simulink model "controller"  (R2019b)
settings: Solver=VariableStepAuto  StartTime=0.0  StopTime=10.0  RelTol=1e-3
settings Model: Creator=Avmash  LastModifiedBy=Avmash

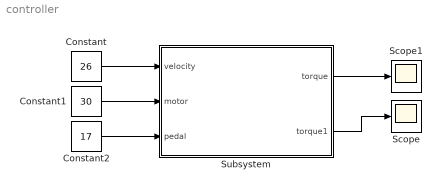
== system controller ==
  Constant : Constant  Value=26
  Constant1 : Constant  Value=30
  Constant2 : Constant  Value=17
  Scope : Scope
  Scope1 : Scope
  Subsystem : Subsystem
  wires:
  Constant/1 -> Subsystem/1(velocity)
  Constant1/1 -> Subsystem/2(motor)
  Subsystem/2(torque1) -> Scope/1
  Subsystem/1(torque) -> Scope1/1
  Constant2/1 -> Subsystem/3(pedal)

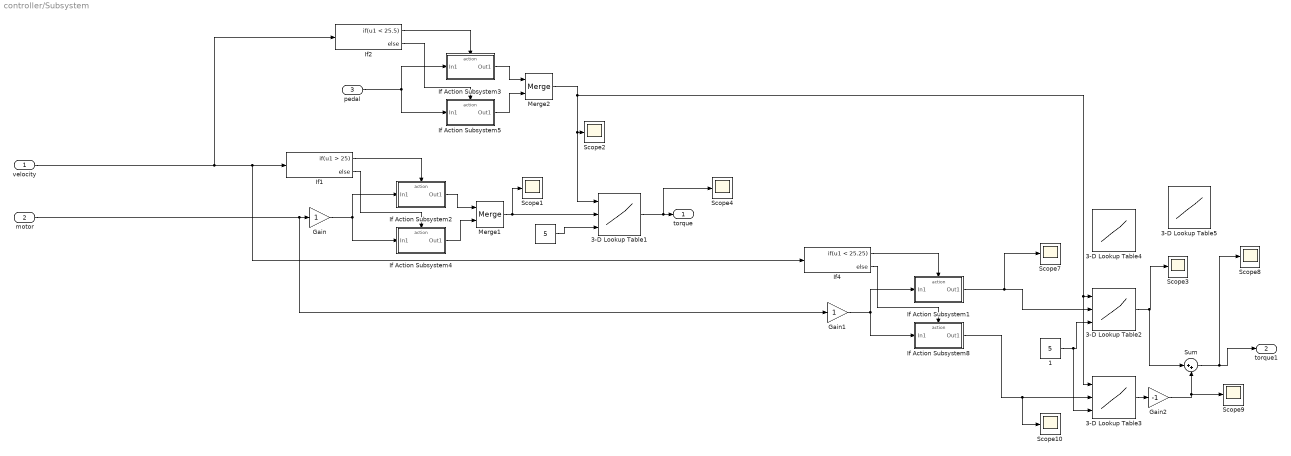
== system controller/Subsystem ==
  velocity : Inport
  motor : Inport  Port=2
  pedal : Inport  Port=3
  " " : Constant  Value=5
  " 1" : Constant  Value=5
  3-D Lookup Table1 : Lookup_n-D  NumberOfTableDimensions=3  BreakpointsForDimension1=[0,5,10,15,20]  BreakpointsForDimension2=[0,10,20,30,40]  BreakpointsForDimension3=[5, 7]  Table=reshape([0,5,10,15,20,0,10,15,20,25,0,10,20,25,30,0,10,20,30,35,0,10,20,30,40,0,5,10,15,20,0,10,15,20,25,0,10,20,25,30,0,10,20,30,35,0,10,20,30,40],5,5,2)  InternalRulePriority=Speed  RndMeth=Simplest  InputSameDT=on
  3-D Lookup Table2 : Lookup_n-D  NumberOfTableDimensions=3  BreakpointsForDimension1=[0,5,10,15,20]  BreakpointsForDimension2=[0,10,20,30,40]  BreakpointsForDimension3=[5, 7]  Table=reshape([0,5,10,15,20,0,10,15,20,25,0,10,20,25,30,0,10,20,30,35,0,10,20,30,40,0,5,10,15,20,0,10,15,20,25,0,10,20,25,30,0,10,20,30,35,0,10,20,30,40],5,5,2)  InternalRulePriority=Speed  RndMeth=Simplest  InputSameDT=on
  3-D Lookup Table3 : Lookup_n-D  NumberOfTableDimensions=3  BreakpointsForDimension1=[0,5,10,15,20]  BreakpointsForDimension2=[0,10,20,30,40]  BreakpointsForDimension3=[5, 7]  Table=reshape([0,0,0,0,0,0,10,15,20,25,0,10,20,25,30,0,10,20,30,35,0,10,20,30,40,0,5,10,15,20,0,10,15,20,25,0,10,20,25,30,0,10,20,30,35,0,10,20,30,40],5,5,2)  InternalRulePriority=Speed  RndMeth=Simplest  InputSameDT=on
  3-D Lookup Table4 : Lookup_n-D  NumberOfTableDimensions=3  BreakpointsForDimension1=[0,5,10,15,20]  BreakpointsForDimension2=[-40,-30,-20,-10,0,10,20,30,40]  BreakpointsForDimension3=[5, 7]  Table=reshape([0,-10,-20,-30,-40,0,-10,-20,-30,-35,0,-10,-20,-25,-30,0,-10,-15,-20,-25,0,5,10,15,20,0,10,15,20,25,0,10,20,25,30,0,10,20,30,35,0,10,20,30,40,0,-10,-20,-30,-40,0,-10,-20,-30,-35,0,-10,-20,-25,-30,0,-10,-15,-20,-25,0,5,10,15,20,0,10,15,20,25,0,10,20,25,30,0,10,20,30,35,0,10,20,30,40],5,9,2)  InternalRulePriority=Speed  RndMeth=Simplest  InputSameDT=on
  3-D Lookup Table5 : Lookup_n-D  NumberOfTableDimensions=3  BreakpointsForDimension1=[0,5,10,15,20]  BreakpointsForDimension2=[-40,-30,-20,-10,0]  BreakpointsForDimension3=[5, 7]  Table=|  InternalRulePriority=Speed  RndMeth=Simplest  InputSameDT=on
      | reshape([
      | 0,-10,-20,-30,-40,0,-10,-20,-30,-35,0,-10,-20,-25,-30,0,-10,-15,-20,-25,0,5,10,15,20,0,-10,-20,-30,-40,0,-10,-20,-30,-35,0,-10,-20,-25,-30,0,-10,-15,-20,-25,0,5,10,15,20],5,5,2)
  Gain : Gain
  Gain1 : Gain
  Gain2 : Gain  Gain=-1
  If Action Subsystem1 : Subsystem  TreatAsAtomicUnit=on
  If Action Subsystem2 : Subsystem  TreatAsAtomicUnit=on
  If Action Subsystem3 : Subsystem  TreatAsAtomicUnit=on
  If Action Subsystem4 : Subsystem  TreatAsAtomicUnit=on
  If Action Subsystem5 : Subsystem  TreatAsAtomicUnit=on
  If Action Subsystem8 : Subsystem  TreatAsAtomicUnit=on
  If1 : If  IfExpression=u1 > 25
  If2 : If  IfExpression=u1 < 25.5
  If4 : If  IfExpression=u1 < 25.25
  Merge1 : Merge
  Merge2 : Merge
  Scope{1..4,7..10} (8 alike) : Scope
  Sum : Sum  Inputs=|++
  torque : Outport
  torque1 : Outport  Port=2
  wires:
  " "/1 -> 3-D Lookup Table1/3
  Gain/1 -> If Action Subsystem2/1(In1), If Action Subsystem4/1(In1)
  3-D Lookup Table1/1 -> Scope4/1, torque/1
  Merge1/1 -> 3-D Lookup Table1/2, Scope1/1
  Merge2/1 -> 3-D Lookup Table3/1, 3-D Lookup Table2/1, Scope2/1, 3-D Lookup Table1/1
  If Action Subsystem4/1(Out1) -> Merge1/2
  If Action Subsystem2/1(Out1) -> Merge1/1
  If Action Subsystem3/1(Out1) -> Merge2/1
  If2/1 -> If Action Subsystem3/Action
  If Action Subsystem5/1(Out1) -> Merge2/2
  If2/2 -> If Action Subsystem5/Action
  If1/1 -> If Action Subsystem2/Action
  If1/2 -> If Action Subsystem4/Action
  motor/1 -> Gain1/1, Gain/1
  3-D Lookup Table2/1 -> Sum/1, Scope3/1
  If4/2 -> If Action Subsystem8/Action
  If4/1 -> If Action Subsystem1/Action
  If Action Subsystem1/1(Out1) -> Scope7/1, 3-D Lookup Table2/2
  If Action Subsystem8/1(Out1) -> 3-D Lookup Table3/2, Scope10/1
  Gain1/1 -> If Action Subsystem8/1(In1), If Action Subsystem1/1(In1)
  " 1"/1 -> 3-D Lookup Table3/3, 3-D Lookup Table2/3
  velocity/1 -> If4/1, If1/1, If2/1
  pedal/1 -> If Action Subsystem3/1(In1), If Action Subsystem5/1(In1)
  3-D Lookup Table3/1 -> Gain2/1
  Sum/1 -> Scope8/1, torque1/1
  Gain2/1 -> Scope9/1, Sum/2

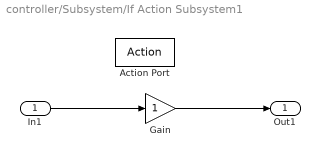
== system controller/Subsystem/If Action Subsystem1 ==
  In1 : Inport
  Action Port : ActionPort  ActionPortLabel=if(u1 < 25.25)
  Gain : Gain
  Out1 : Outport
  wires:
  In1/1 -> Gain/1
  Gain/1 -> Out1/1

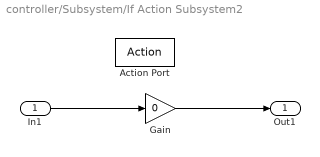
== system controller/Subsystem/If Action Subsystem2 ==
  In1 : Inport
  Action Port : ActionPort  ActionPortLabel=if(u1 > 25)
  Gain : Gain  Gain=0
  Out1 : Outport
  wires:
  Gain/1 -> Out1/1
  In1/1 -> Gain/1

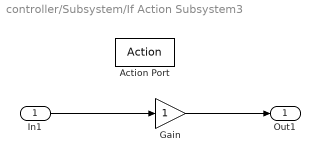
== system controller/Subsystem/If Action Subsystem3 ==
  In1 : Inport
  Action Port : ActionPort  ActionPortLabel=if(u1 < 25.5)
  Gain : Gain
  Out1 : Outport
  wires:
  Gain/1 -> Out1/1
  In1/1 -> Gain/1

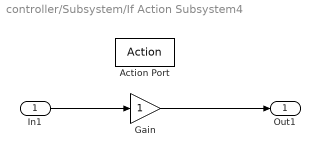
== system controller/Subsystem/If Action Subsystem4 ==
  In1 : Inport
  Action Port : ActionPort  ActionPortLabel=else
  Gain : Gain
  Out1 : Outport
  wires:
  In1/1 -> Gain/1
  Gain/1 -> Out1/1

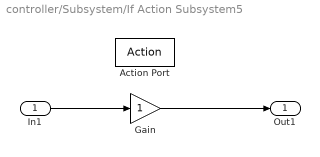
== system controller/Subsystem/If Action Subsystem5 ==
  In1 : Inport
  Action Port : ActionPort  ActionPortLabel=else
  Gain : Gain
  Out1 : Outport
  wires:
  In1/1 -> Gain/1
  Gain/1 -> Out1/1

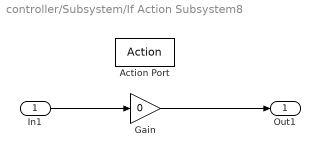
== system controller/Subsystem/If Action Subsystem8 ==
  In1 : Inport
  Action Port : ActionPort  ActionPortLabel=else
  Gain : Gain  Gain=0
  Out1 : Outport
  wires:
  Gain/1 -> Out1/1
  In1/1 -> Gain/1
